simulink model "Assignment_2_3K04"  (R2022b)
settings: Solver=FixedStepAuto  StartTime=0.0  StopTime=1  FixedStep=1e-3  RelTol=1e-3  EnableMultiTasking=on
undefined symbols (not defined in the file): A0, A1, D0, D1, D10, D11, D12, D13, D2, D3, D4, D5, D6, D7, D8, D9, PTA0, PTA1, PTA2, PTB2, PTB23, PTB3, PTB9, PTC16, PTC17, PTC2, PTC3, PTC4, PTD0, PTD1, PTD2, PTD3
libraries: frdmk64flib x19, dspstat3 x1
settings Model: ExtModeTrigDuration=5  Creator=Stephen Oh  LastModifiedBy=Mehak
settings SolverCC: AlgebraicLoopSolver=TrustRegion
settings OptimizationCC: EnhancedBackFolding=on  PassReuseOutputArgsAs=Individual arguments  ZeroExternalMemoryAtStartup=off  ZeroInternalMemoryAtStartup=off  MaxStackSize=64  OptimizeBlockOrder=speed  DifferentSizesBufferReuse=on  OptimizationCustomize=off  EfficientTunableParamExpr=on
settings DebuggingCC: ParameterTunabilityLossMsg=error  UnconnectedInputMsg=warning  UnconnectedOutputMsg=warning  UnconnectedLineMsg=warning  SFMachineParentedDataDiag=warning
settings HardwareCC: ProdBitPerPointer=32  ProdBitPerSizeT=32  ProdBitPerPtrDiffT=32  ProdLargestAtomicInteger=Long  ProdLargestAtomicFloat=Double  ProdWordSize=32  ProdHWDeviceType=ARM Compatible->ARM Cortex
settings ModelReferenceCC: EnableRefExpFcnMdlSchedulingChecks=on
settings SFSimCC: MATLABDynamicMemAlloc=off
settings RTWCC: Description=Embedded Coder  SystemTargetFile=ert.tlc  HardwareBoard=NXP FRDM-K64F  TLCOptions="-aInlineSetEventsForThisBaseRateFcn=TLC_FALSE -aSuppressMultiTaskScheduler=TLC_FALSE  -aRateBasedStepFcn=0"  TemplateMakefile=ert_default_tmf  Toolchain=GNU Tools for ARM Embedded Processors
settings CodeAppCC: ForceParamTrailComments=on  IgnoreCustomStorageClasses=off  OperatorAnnotations=on  SimulinkDataObjDesc=on  SFDataObjDesc=on  InsertBlockDesc=on

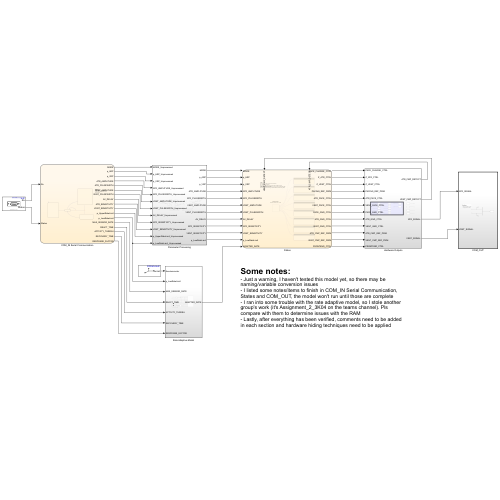
[thumbnail: Simulink's stored preview of the top-level diagram]
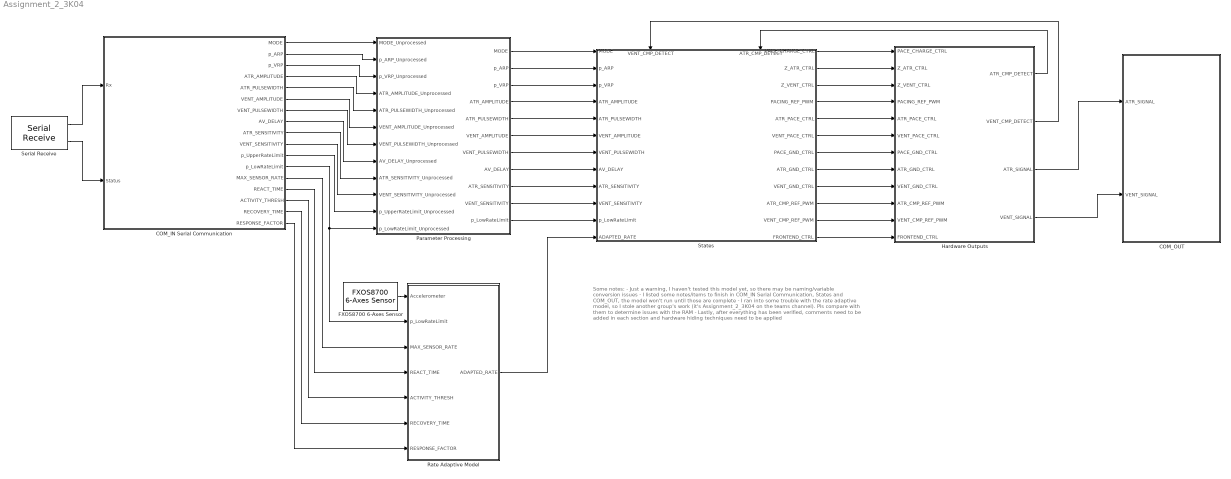
== system Assignment_2_3K04 ==
  note: Some notes:
      | - Just a warning, I haven't tested this model yet, so there may be naming/variable conversion issues
      | - I listed some notes/items to finish in COM_IN Serial Communication, States and COM_OUT, the model won't run until those are complete
      | - I ran into some trouble with the rate adaptive model, so I stole another group's work (it's Assignment_2_3K04 on the teams channel). Pls compare with them to determine issues with the RAM
      | - Lastly, after everything has been verified, comments need to be added in each section and hardware hiding techniques need to be applied
  " States" : Stateflow chart  TreatAsAtomicUnit=on
      settings: PortSchema="{\"entries\":[{\"content\":{\"sides\":[{\"content\":{\"connectorIds\":[\"In1\",\"In4\",\"In5\",\"In6\",\"In7\",\"In11\",\"In12\",\"In14\",\"In9\",\"In10\",\"In8\",\"In13\"]},\"type\":\"ConnectorPlacement.EquallySpacedRectSide\",\"uuid\":\"15e03f69-5c25-4f3e-b3fb-d71978e552f4\"},{\"content\":{\"connectorIds\":[\"Out7\",\"Out4\",\"Out5\",\"Out8\",\"Out9\",\"Out3\",\"Out6\",\"Out1\",\"Out2\",\"Out10\",\"Out12\",\"Out11\"],\"side\":\"RIGHT\"},\"type\":\"ConnectorPlacement.EquallySpacedRectSide\",\"uuid\":\"02171bf1-edb1-4b01-9e56-a8642c556ed6\"},{\"content\":{\"connectorIds\":[\"In3\",\"In2\"],\"side\":\"TOP\"},\"type\":\"ConnectorPlacement.EquallySpacedRectSide\",\"uuid\":\"cc6b5506-3435-4740-9e3f-4dfe15d30bff\"}]},\"type\":\"ConnectorPlacement.EquallySpacedConnector\",\"uuid\":\"0ad55da7-1e65-48d0-a0a4-2620ffa94320\"}],\"packageUris\":[\"http://schema.mathworks.com/mf0/Connector/R2020b\"],\"version\":\"1.0\"}"
  COM_IN Serial Communication : Stateflow chart  TreatAsAtomicUnit=on
      settings: PortSchema="{\"entries\":[{\"content\":{\"sides\":[{\"content\":{\"connectorIds\":[\"In1\",\"In2\"]},\"type\":\"ConnectorPlacement.EquallySpacedRectSide\",\"uuid\":\"22fa9edc-2a49-4280-8e8e-0842a45ddb47\"},{\"content\":{\"connectorIds\":[\"Out1\",\"Out2\",\"Out5\",\"Out6\",\"Out9\",\"Out7\",\"Out8\",\"Out11\",\"Out17\",\"Out12\",\"Out4\",\"Out3\",\"Out10\",\"Out13\",\"Out14\",\"Out16\",\"Out15\"],\"side\":\"RIGHT\"},\"type\":\"ConnectorPlacement.EquallySpacedRectSide\",\"uuid\":\"653d204d-01e6-4b1d-8e7b-47ebaddcd032\"},{\"content\":{\"connectorIds\":[],\"side\":\"TOP\"},\"type\":\"ConnectorPlacement.EquallySpacedRectSide\",\"uuid\":\"5fb759fd-937e-492d-8a65-272e5a7048d8\"}]},\"type\":\"ConnectorPlacement.EquallySpacedConnector\",\"uuid\":\"8ef65fa3-58c0-4e1e-983b-59a6af0cca9a\"}],\"packageUris\":[\"http://schema.mathworks.com/mf0/Connector/R2020b\"],\"version\":\"1.0\"}"
  COM_OUT : Subsystem  TreatAsAtomicUnit=on
  FXOS8700 6-Axes Sensor : frdmk64flib/FXOS8700 6-Axes Sensor  Activesensor=Accelerometer only  ODR=800Hz  HybridODR=400Hz  Accelfullrange=-4g to +4g  SampleTime=-1
  Hardware Outputs : Subsystem
  Parameter Processing : Subsystem
  Rate Adaptive Model : Subsystem
  Serial Receive : frdmk64flib/Serial Receive  SCIModule=0  Baudrate=uint32(9600)  Parity=None  StopBits=1  HardwareFlowControl=None  ByteOrder=LittleEndian  DataType=uint8  DataLength=34  BlockingMode=off  OutputStatus=on  SampleTime=0.1
  wires:
  " States"/7(PACE_CHARGE_CTRL) -> Hardware Outputs/1(PACE_CHARGE_CTRL)
  " States"/4(Z_ATR_CTRL) -> Hardware Outputs/2(Z_ATR_CTRL)
  " States"/5(Z_VENT_CTRL) -> Hardware Outputs/3(Z_VENT_CTRL)
  " States"/8(PACING_REF_PWM) -> Hardware Outputs/4(PACING_REF_PWM)
  " States"/9(ATR_PACE_CTRL) -> Hardware Outputs/5(ATR_PACE_CTRL)
  " States"/3(VENT_PACE_CTRL) -> Hardware Outputs/6(VENT_PACE_CTRL)
  " States"/6(PACE_GND_CTRL) -> Hardware Outputs/7(PACE_GND_CTRL)
  " States"/1(ATR_GND_CTRL) -> Hardware Outputs/8(ATR_GND_CTRL)
  " States"/2(VENT_GND_CTRL) -> Hardware Outputs/9(VENT_GND_CTRL)
  " States"/10(ATR_CMP_REF_PWM) -> Hardware Outputs/10(ATR_CMP_REF_PWM)
  " States"/12(VENT_CMP_REF_PWM) -> Hardware Outputs/11(VENT_CMP_REF_PWM)
  " States"/11(FRONTEND_CTRL) -> Hardware Outputs/12(FRONTEND_CTRL)
  Serial Receive/1 -> COM_IN Serial Communication/1(Rx)
  Serial Receive/2 -> COM_IN Serial Communication/2(Status)
  Hardware Outputs/1(ATR_CMP_DETECT) -> " States"/2(ATR_CMP_DETECT)
  Hardware Outputs/2(VENT_CMP_DETECT) -> " States"/3(VENT_CMP_DETECT)
  FXOS8700 6-Axes Sensor/1 -> Rate Adaptive Model/1(Accelerometer)
  COM_IN Serial Communication/3(p_LowRateLimit) -> Rate Adaptive Model/2(p_LowRateLimit), Parameter Processing/12(p_LowRateLimit_Unprocessed)
  COM_IN Serial Communication/10(MAX_SENSOR_RATE) -> Rate Adaptive Model/3(MAX_SENSOR_RATE)
  COM_IN Serial Communication/13(REACT_TIME) -> Rate Adaptive Model/4(REACT_TIME)
  COM_IN Serial Communication/14(ACTIVITY_THRESH) -> Rate Adaptive Model/5(ACTIVITY_THRESH)
  COM_IN Serial Communication/15(RESPONSE_FACTOR) -> Rate Adaptive Model/7(RESPONSE_FACTOR)
  COM_IN Serial Communication/16(RECOVERY_TIME) -> Rate Adaptive Model/6(RECOVERY_TIME)
  COM_IN Serial Communication/4(p_UpperRateLimit) -> Parameter Processing/11(p_UpperRateLimit_Unprocessed)
  COM_IN Serial Communication/17(ATR_SENSITIVITY) -> Parameter Processing/9(ATR_SENSITIVITY_Unprocessed)
  COM_IN Serial Communication/12(VENT_SENSITIVITY) -> Parameter Processing/10(VENT_SENSITIVITY_Unprocessed)
  COM_IN Serial Communication/6(ATR_AMPLITUDE) -> Parameter Processing/4(ATR_AMPLITUDE_Unprocessed)
  COM_IN Serial Communication/7(VENT_AMPLITUDE) -> Parameter Processing/6(VENT_AMPLITUDE_Unprocessed)
  COM_IN Serial Communication/1(MODE) -> Parameter Processing/1(MODE_Unprocessed)
  COM_IN Serial Communication/2(p_ARP) -> Parameter Processing/2(p_ARP_Unprocessed)
  COM_IN Serial Communication/5(p_VRP) -> Parameter Processing/3(p_VRP_Unprocessed)
  COM_IN Serial Communication/9(ATR_PULSEWIDTH) -> Parameter Processing/5(ATR_PULSEWIDTH_Unprocessed)
  COM_IN Serial Communication/8(VENT_PULSEWIDTH) -> Parameter Processing/7(VENT_PULSEWIDTH_Unprocessed)
  COM_IN Serial Communication/11(AV_DELAY) -> Parameter Processing/8(AV_DELAY_Unprocessed)
  Parameter Processing/1(MODE) -> " States"/1(MODE)
  Parameter Processing/2(p_ARP) -> " States"/4(p_ARP)
  Parameter Processing/3(p_VRP) -> " States"/5(p_VRP)
  Parameter Processing/11(p_LowRateLimit) -> " States"/8(p_LowRateLimit)
  Parameter Processing/10(VENT_SENSITIVITY) -> " States"/10(VENT_SENSITIVITY)
  Parameter Processing/9(ATR_SENSITIVITY) -> " States"/9(ATR_SENSITIVITY)
  Parameter Processing/4(ATR_AMPLITUDE) -> " States"/6(ATR_AMPLITUDE)
  Parameter Processing/5(ATR_PULSEWIDTH) -> " States"/7(ATR_PULSEWIDTH)
  Parameter Processing/6(VENT_AMPLITUDE) -> " States"/11(VENT_AMPLITUDE)
  Parameter Processing/7(VENT_PULSEWIDTH) -> " States"/12(VENT_PULSEWIDTH)
  Rate Adaptive Model/1(ADAPTED_RATE) -> " States"/13(ADAPTED_RATE)
  Parameter Processing/8(AV_DELAY) -> " States"/14(AV_DELAY)
  Hardware Outputs/3(ATR_SIGNAL) -> COM_OUT/1(ATR_SIGNAL)
  Hardware Outputs/4(VENT_SIGNAL) -> COM_OUT/2(VENT_SIGNAL)

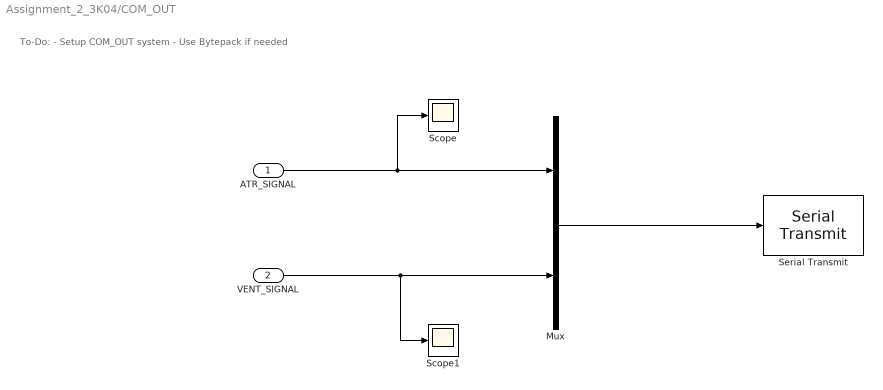
== system Assignment_2_3K04/COM_OUT ==
  note: To-Do:
      | - Setup COM_OUT system
      | - Use Bytepack if needed
  ATR_SIGNAL : Inport  OutDataTypeStr=double
  VENT_SIGNAL : Inport  Port=2  OutDataTypeStr=double
  Mux : Mux  Inputs=2
  Scope : Scope
  Scope1 : Scope
  Serial Transmit : frdmk64flib/Serial Transmit  SCIModule=0  Baudrate=uint32(9600)  Parity=None  StopBits=1  HardwareFlowControl=None  ByteOrder=LittleEndian  BlockingMode=on  OutputStatus=off
  wires:
  ATR_SIGNAL/1 -> Scope/1, Mux/1
  Mux/1 -> Serial Transmit/1
  VENT_SIGNAL/1 -> Scope1/1, Mux/2

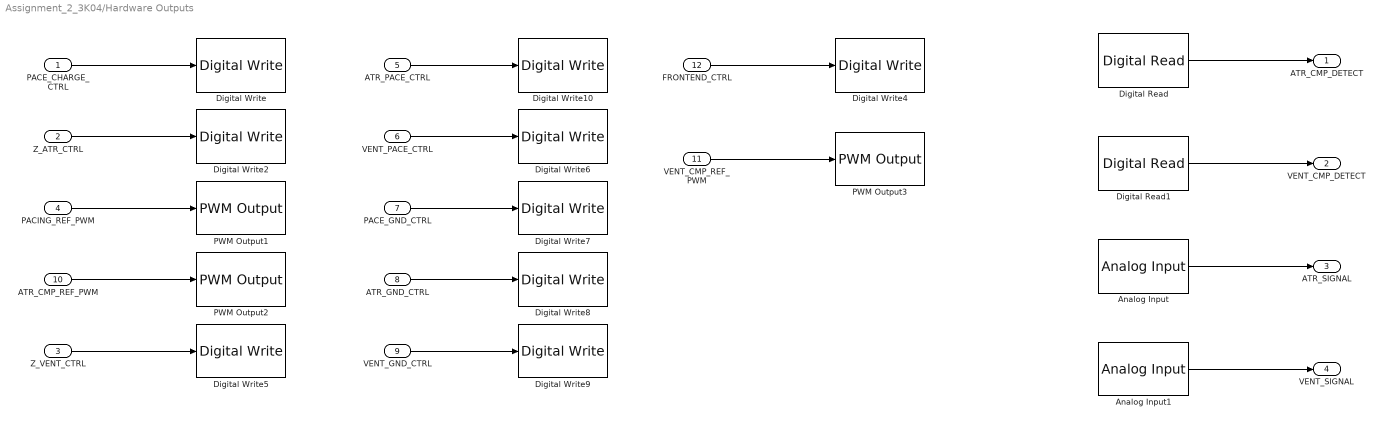
== system Assignment_2_3K04/Hardware Outputs ==
  PACE_CHARGE_CTRL : Inport
  Z_ATR_CTRL : Inport  Port=2
  Z_VENT_CTRL : Inport  Port=3
  PACING_REF_PWM : Inport  Port=4
  ATR_PACE_CTRL : Inport  Port=5
  VENT_PACE_CTRL : Inport  Port=6
  PACE_GND_CTRL : Inport  Port=7
  ATR_GND_CTRL : Inport  Port=8
  VENT_GND_CTRL : Inport  Port=9
  ATR_CMP_REF_PWM : Inport  Port=10
  VENT_CMP_REF_PWM : Inport  Port=11
  FRONTEND_CTRL : Inport  Port=12
  Analog Input : frdmk64flib/Analog Input  Whichpin=PTB2 (A0)  SampleTime=-1
  Analog Input1 : frdmk64flib/Analog Input  Whichpin=PTB3 (A1)  SampleTime=-1
  Digital Read : frdmk64flib/Digital Read  Whichpin=PTC16 (D0)  SampleTime=-1
  Digital Read1 : frdmk64flib/Digital Read  Whichpin=PTC17 (D1)  SampleTime=-1
  Digital Write : frdmk64flib/Digital Write  Whichpin=PTB9 (D2)
  Digital Write10 : frdmk64flib/Digital Write  Whichpin=PTA0 (D8)
  Digital Write2 : frdmk64flib/Digital Write  Whichpin=PTB23 (D4)
  Digital Write4 : frdmk64flib/Digital Write  Whichpin=PTD1 (D13)
  Digital Write5 : frdmk64flib/Digital Write  Whichpin=PTC3 (D7)
  Digital Write6 : frdmk64flib/Digital Write  Whichpin=PTC4 (D9)
  Digital Write7 : frdmk64flib/Digital Write  Whichpin=PTD0 (D10)
  Digital Write8 : frdmk64flib/Digital Write  Whichpin=PTD2 (D11)
  Digital Write9 : frdmk64flib/Digital Write  Whichpin=PTD3 (D12)
  PWM Output1 : frdmk64flib/PWM Output  Whichpin=PTA2 (D5)  InitialFrequency=2000  InitialDutyCycle=0
  PWM Output2 : frdmk64flib/PWM Output  Whichpin=PTC2 (D6)  InitialFrequency=2000  InitialDutyCycle=0
  PWM Output3 : frdmk64flib/PWM Output  Whichpin=PTA1 (D3)  InitialFrequency=2000  InitialDutyCycle=0
  ATR_CMP_DETECT : Outport
  VENT_CMP_DETECT : Outport  Port=2
  ATR_SIGNAL : Outport  Port=3  OutDataTypeStr=double
  VENT_SIGNAL : Outport  Port=4  OutDataTypeStr=double
  wires:
  ATR_GND_CTRL/1 -> Digital Write8/1
  Z_ATR_CTRL/1 -> Digital Write2/1
  VENT_PACE_CTRL/1 -> Digital Write6/1
  PACING_REF_PWM/1 -> PWM Output1/1
  VENT_GND_CTRL/1 -> Digital Write9/1
  PACE_GND_CTRL/1 -> Digital Write7/1
  FRONTEND_CTRL/1 -> Digital Write4/1
  PACE_CHARGE_CTRL/1 -> Digital Write/1
  Z_VENT_CTRL/1 -> Digital Write5/1
  ATR_CMP_REF_PWM/1 -> PWM Output2/1
  ATR_PACE_CTRL/1 -> Digital Write10/1
  VENT_CMP_REF_PWM/1 -> PWM Output3/1
  Digital Read/1 -> ATR_CMP_DETECT/1
  Digital Read1/1 -> VENT_CMP_DETECT/1
  Analog Input/1 -> ATR_SIGNAL/1
  Analog Input1/1 -> VENT_SIGNAL/1

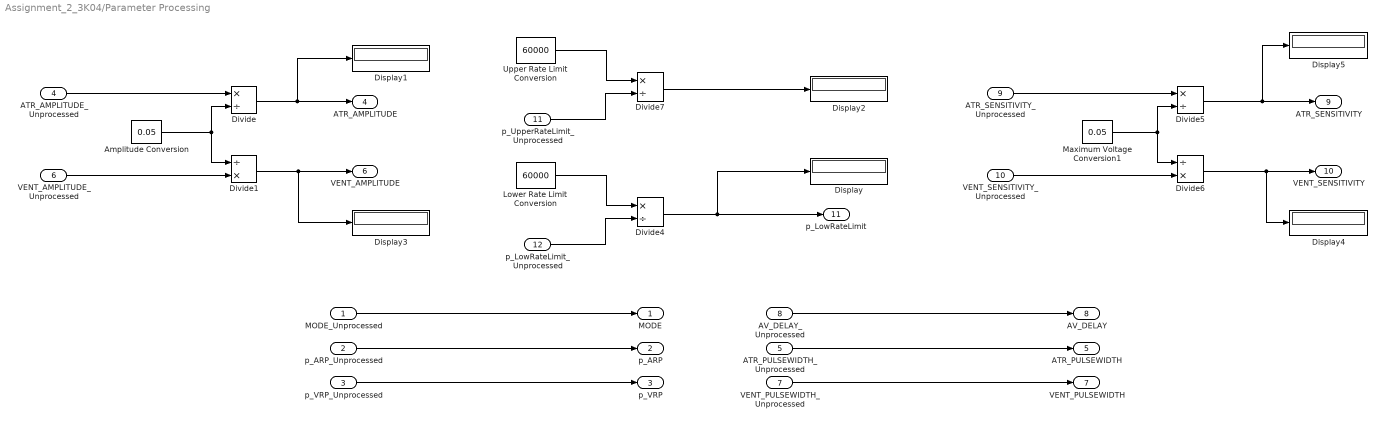
== system Assignment_2_3K04/Parameter Processing ==
  MODE_Unprocessed : Inport  OutDataTypeStr=single
  p_ARP_Unprocessed : Inport  Port=2  OutDataTypeStr=single
  p_VRP_Unprocessed : Inport  Port=3  OutDataTypeStr=single
  ATR_AMPLITUDE_Unprocessed : Inport  Port=4  OutDataTypeStr=single
  ATR_PULSEWIDTH_Unprocessed : Inport  Port=5  OutDataTypeStr=single
  VENT_AMPLITUDE_Unprocessed : Inport  Port=6  OutDataTypeStr=single
  VENT_PULSEWIDTH_Unprocessed : Inport  Port=7  OutDataTypeStr=single
  AV_DELAY_Unprocessed : Inport  Port=8  OutDataTypeStr=single
  ATR_SENSITIVITY_Unprocessed : Inport  Port=9  OutDataTypeStr=single
  VENT_SENSITIVITY_Unprocessed : Inport  Port=10  OutDataTypeStr=single
  p_UpperRateLimit_Unprocessed : Inport  Port=11
  p_LowRateLimit_Unprocessed : Inport  Port=12
  Amplitude Conversion : Constant  Value=0.05
  Display{,1..5} (6 alike) : Display
  Divide : Product  Inputs=*/  OutDataTypeStr=uint8
  Divide1 : Product  Inputs=/*  OutDataTypeStr=uint8
  Divide4 : Product  Inputs=*/  OutDataTypeStr=Inherit: Keep MSB  RndMeth=Nearest
  Divide5 : Product  Inputs=*/  OutDataTypeStr=uint8
  Divide6 : Product  Inputs=/*  OutDataTypeStr=uint8
  Divide7 : Product  Inputs=*/  OutDataTypeStr=Inherit: Keep MSB  RndMeth=Nearest
  Lower Rate Limit Conversion : Constant  Value=60000
  Maximum Voltage Conversion1 : Constant  Value=0.05
  Upper Rate Limit Conversion : Constant  Value=60000
  MODE : Outport
  p_ARP : Outport  Port=2
  p_VRP : Outport  Port=3
  ATR_AMPLITUDE : Outport  Port=4  OutDataTypeStr=uint8
  ATR_PULSEWIDTH : Outport  Port=5
  VENT_AMPLITUDE : Outport  Port=6  OutDataTypeStr=uint8
  VENT_PULSEWIDTH : Outport  Port=7
  AV_DELAY : Outport  Port=8
  ATR_SENSITIVITY : Outport  Port=9  OutDataTypeStr=uint8
  VENT_SENSITIVITY : Outport  Port=10  OutDataTypeStr=uint8
  p_LowRateLimit : Outport  Port=11
  wires:
  Amplitude Conversion/1 -> Divide1/1, Divide/2
  ATR_AMPLITUDE_Unprocessed/1 -> Divide/1
  VENT_AMPLITUDE_Unprocessed/1 -> Divide1/2
  Divide/1 -> Display1/1, ATR_AMPLITUDE/1
  Divide1/1 -> Display3/1, VENT_AMPLITUDE/1
  Divide6/1 -> Display4/1, VENT_SENSITIVITY/1
  Maximum Voltage Conversion1/1 -> Divide6/1, Divide5/2
  ATR_SENSITIVITY_Unprocessed/1 -> Divide5/1
  Divide5/1 -> Display5/1, ATR_SENSITIVITY/1
  VENT_SENSITIVITY_Unprocessed/1 -> Divide6/2
  Divide4/1 -> p_LowRateLimit/1, Display/1
  p_LowRateLimit_Unprocessed/1 -> Divide4/2
  Lower Rate Limit Conversion/1 -> Divide4/1
  Divide7/1 -> Display2/1
  Upper Rate Limit Conversion/1 -> Divide7/1
  p_UpperRateLimit_Unprocessed/1 -> Divide7/2
  MODE_Unprocessed/1 -> MODE/1
  p_ARP_Unprocessed/1 -> p_ARP/1
  p_VRP_Unprocessed/1 -> p_VRP/1
  VENT_PULSEWIDTH_Unprocessed/1 -> VENT_PULSEWIDTH/1
  AV_DELAY_Unprocessed/1 -> AV_DELAY/1
  ATR_PULSEWIDTH_Unprocessed/1 -> ATR_PULSEWIDTH/1

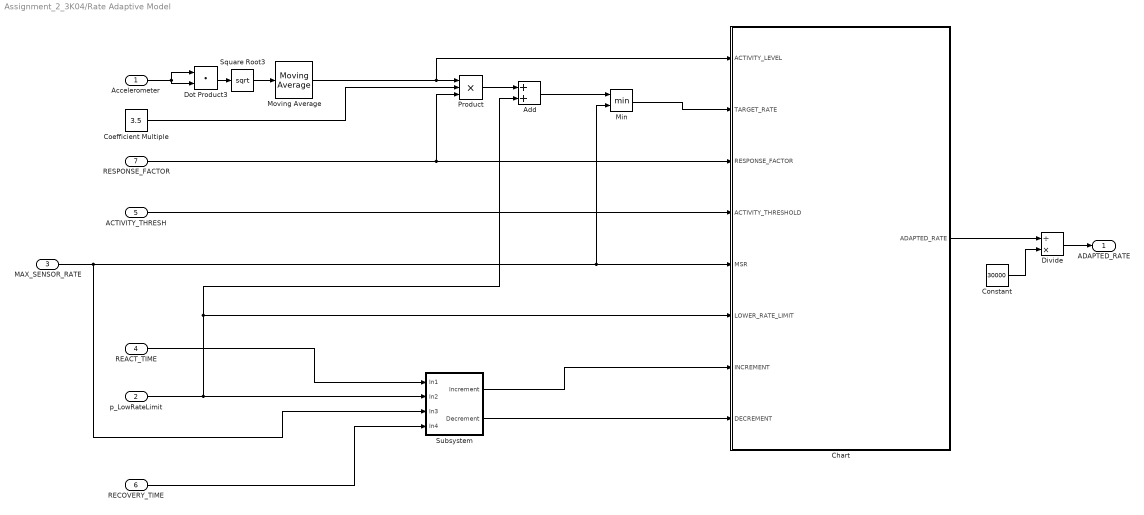
== system Assignment_2_3K04/Rate Adaptive Model ==
  Accelerometer : Inport
  p_LowRateLimit : Inport  Port=2
  MAX_SENSOR_RATE : Inport  Port=3
  REACT_TIME : Inport  Port=4
  ACTIVITY_THRESH : Inport  Port=5
  RECOVERY_TIME : Inport  Port=6
  RESPONSE_FACTOR : Inport  Port=7
  Add : Sum
  Chart : Stateflow chart  TreatAsAtomicUnit=on
      settings: PortSchema="{\"entries\":[{\"content\":{\"sides\":[{\"content\":{\"connectorIds\":[\"In1\",\"In3\",\"In2\",\"In6\",\"In8\",\"In7\",\"In4\",\"In5\"]},\"type\":\"ConnectorPlacement.EquallySpacedRectSide\",\"uuid\":\"efebee7e-2c09-4b25-ba04-904f72c011ed\"},{\"content\":{\"connectorIds\":[\"Out1\"],\"side\":\"RIGHT\"},\"type\":\"ConnectorPlacement.EquallySpacedRectSide\",\"uuid\":\"6322cc63-1b7a-423a-b49b-7b27e71e0c32\"},{\"content\":{\"connectorIds\":[],\"side\":\"TOP\"},\"type\":\"ConnectorPlacement.EquallySpacedRectSide\",\"uuid\":\"daf2dbd4-7676-46e9-bb01-958bd0e2e14e\"}]},\"type\":\"ConnectorPlacement.EquallySpacedConnector\",\"uuid\":\"43c3c7b3-b94c-45f5-b310-1a430cfb2b71\"}],\"packageUris\":[\"http://schema.mathworks.com/mf0/Connector/19700101\"],\"version\":\"1.0\"}"
  Coefficient Multiple : Constant  Value=3.5
  Constant : Constant  Value=30000
  Divide : Product  Inputs=/*
  Dot Product3 : DotProduct  OutDataTypeStr=Inherit: Inherit via internal rule
  Min : MinMax  Inputs=2
  Moving Average : dspstat3/Moving Average  Method=Sliding window  ForgettingFactorPort=off  SpecifyWindowLength=on  WindowLength=500  OverlapLength=499  AllowArbitraryInputLength=off  ForgettingFactor=0.9  SimulateUsing=Code generation
  Product : Product  Inputs=3
  Square Root3 : Sqrt
  Subsystem : Subsystem
  ADAPTED_RATE : Outport
  wires:
  RECOVERY_TIME/1 -> Subsystem/4(In4)
  MAX_SENSOR_RATE/1 -> Subsystem/3(In3), Min/2, Chart/8(MSR)
  Subsystem/1(Increment) -> Chart/4(INCREMENT)
  ACTIVITY_THRESH/1 -> Chart/6(ACTIVITY_THRESHOLD)
  RESPONSE_FACTOR/1 -> Product/3, Chart/2(RESPONSE_FACTOR)
  p_LowRateLimit/1 -> Subsystem/2(In2), Chart/7(LOWER_RATE_LIMIT), Add/2
  Add/1 -> Min/1
  Product/1 -> Add/1
  Min/1 -> Chart/3(TARGET_RATE)
  REACT_TIME/1 -> Subsystem/1(In1)
  Subsystem/2(Decrement) -> Chart/5(DECREMENT)
  Chart/1(ADAPTED_RATE) -> Divide/1
  Coefficient Multiple/1 -> Product/2
  Divide/1 -> ADAPTED_RATE/1
  Constant/1 -> Divide/2
  Moving Average/1 -> Chart/1(ACTIVITY_LEVEL), Product/1
  Square Root3/1 -> Moving Average/1
  Dot Product3/1 -> Square Root3/1
  Accelerometer/1 -> Dot Product3/1, Dot Product3/2

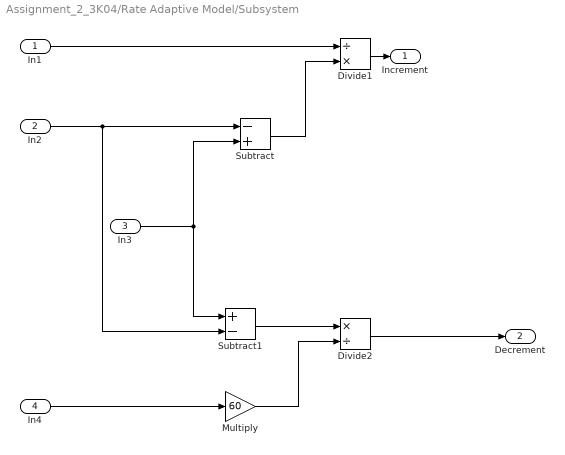
== system Assignment_2_3K04/Rate Adaptive Model/Subsystem ==
  In1 : Inport
  In2 : Inport  Port=2
  In3 : Inport  Port=3
  In4 : Inport  Port=4
  Divide1 : Product  Inputs=/*  OutDataTypeStr=uint8  RndMeth=Ceiling
  Divide2 : Product  Inputs=*/  OutDataTypeStr=uint8  RndMeth=Ceiling  SaturateOnIntegerOverflow=on
  Multiply : Gain  Gain=60
  Subtract : Sum  Inputs=-+
  Subtract1 : Sum  Inputs=+-
  Increment : Outport
  Decrement : Outport  Port=2
  wires:
  Multiply/1 -> Divide2/2
  In2/1 -> Subtract1/2, Subtract/1
  In3/1 -> Subtract/2, Subtract1/1
  Divide1/1 -> Increment/1
  In1/1 -> Divide1/1
  Subtract1/1 -> Divide2/1
  Subtract/1 -> Divide1/2
  In4/1 -> Multiply/1
  Divide2/1 -> Decrement/1

== stateflow chart Assignment_2_3K04/COM_IN Serial Communication ==
  state SET_PARAM
    % Uses serial input to assign values to the parameters
    entry:
    MODE = Rx();
    p_LowRateLimit = Rx();
    p_UpperRateLimit = Rx();
    ATR_AMPLITUDE = Rx();
    VENT_AMPLITUDE = Rx();
    ATR_PULSEWIDTH = Rx();
    VENT_PULSEWIDTH = Rx();
    p_ARP = Rx();
    p_VRP = Rx();
    ATR_SENSITIVITY = Rx();
    VENT_SENSITIVITY = Rx();
    MAX_SENSOR_RATE = Rx();
    RECOVERY_TIME = Rx();
    REACT_TIME = Rx();
    RESPONSE_FACTOR = Rx();
    ACTIVITY_THRESH = Rx();
    AV_DELAY = Rx();
  note: To-Do:
      | - Set number of transmitted bytes
      | - Update SET_PARAM with values
      | - Verify Fuction
  state INITIAL
    % Set the initial values of parameters
    entry:
    MODE = 1;
    p_ARP = 250;
    p_VRP = 320;
    p_LowRateLimit = 60;
    p_UpperRateLimit = 120;
    MAX_SENSOR_RATE = 120;
    ATR_AMPLITUDE = 3.5;
    ATR_PULSEWIDTH = 1;
    VENT_AMPLITUDE = 3.5;
    VENT_PULSEWIDTH = 1;
    AV_DELAY = 150;
    ATR_SENSITIVITY = 4;
    VENT_SENSITIVITY = 4;
    REACT_TIME = 30;
    ACTIVITY_THRESH = 1.1;
    RESPONSE_FACTOR = 8;
    RECOVERY_TIME = 5;
  state STANDBY
    % Wait for COM
  state ECHO_PARAM
    % Sends back the current value of the parameters
    entry:
    send_params()
  (default) -> INITIAL
  SET_PARAM -> STANDBY
  (junction 13) -> SET_PARAM [order 1] : [Rx(2) == hex2dec('55')]
  (junction 12) -> STANDBY [order 2]
  INITIAL -> STANDBY
  STANDBY -> (junction 12) : [Status==0]
  (junction 12) -> (junction 13) [order 1] : [Rx(1) == hex2dec('16')]
  (junction 13) -> ECHO_PARAM [order 2] : [Rx(2) == hex2dec('22')]
  ECHO_PARAM -> STANDBY
  data: Rx input uint8; Status input uint8; MODE output uint8; p_ARP output uint16; p_LowRateLimit output uint8; p_UpperRateLimit output uint8; p_VRP output uint16; ATR_AMPLITUDE output single; VENT_AMPLITUDE output single; VENT_PULSEWIDTH output uint8; ATR_PULSEWIDTH output uint8; MAX_SENSOR_RATE output uint8; AV_DELAY output uint16; VENT_SENSITIVITY output single; REACT_TIME output uint8; ACTIVITY_THRESH output single; RESPONSE_FACTOR output uint8; RECOVERY_TIME output uint8; ATR_SENSITIVITY output single

== stateflow chart Assignment_2_3K04/Rate Adaptive Model/Chart ==
  state RateSelect
    entry:
    ADAPTED_RATE = LOWER_RATE_LIMIT
  state Increment
    entry:
    ADAPTED_RATE = ADAPTED_RATE + INCREMENT
  state TargetRateAchieved
  state Decrement
    entry:
    ADAPTED_RATE = ADAPTED_RATE - DECREMENT
  Increment -> Increment [order 2] : after(1000, msec) [ACTIVITY_LEVEL > ACTIVITY_THRESHOLD]
  (default) -> RateSelect
  Increment -> TargetRateAchieved [order 1] : [ADAPTED_RATE >= TARGET_RATE ]
  RateSelect -> Increment [order 1] : [ACTIVITY_LEVEL > ACTIVITY_THRESHOLD]
  RateSelect -> RateSelect [order 2] : [ACTIVITY_LEVEL < ACTIVITY_THRESHOLD]
  Decrement -> RateSelect [order 3] : [ADAPTED_RATE <= LOWER_RATE_LIMIT]
  Decrement -> Increment [order 1] : after(1000, msec) [ACTIVITY_LEVEL > ACTIVITY_THRESHOLD]
  Increment -> Decrement [order 3] : after(1000, msec) [ACTIVITY_LEVEL < ACTIVITY_THRESHOLD]
  TargetRateAchieved -> Decrement : [ACTIVITY_LEVEL < ACTIVITY_THRESHOLD]
  Decrement -> Decrement [order 2] : after(1000, msec) [ACTIVITY_LEVEL < ACTIVITY_THRESHOLD]
  data: ACTIVITY_LEVEL input; RESPONSE_FACTOR input; ADAPTED_RATE output; TARGET_RATE input; INCREMENT input; DECREMENT input; ACTIVITY_THRESHOLD input; LOWER_RATE_LIMIT input; MSR input

== stateflow chart Assignment_2_3K04/ States ==
  state AOO [group]
    state Charging
      entry:
      %charging capacitor C22
      ATR_PACE_CTRL = 0;
      VENT_PACE_CTRL = 0;
      PACING_REF_PWM = ATR_AMPLITUDE;
      PACE_CHARGE_CTRL = 1;
    state Pacing
      entry:
      %charge release of capacitor C22 into C21
      PACE_CHARGE_CTRL = 0;
      PACE_GND_CTRL = 1;
      ATR_PACE_CTRL = 1;
      ATR_GND_CTRL = 0;
      Z_ATR_CTRL = 0;
      Z_VENT_CTRL = 0;
      VENT_GND_CTRL = 0;
      VENT_PACE_CTRL = 0;
    state Discharging
      entry:
      %charging release of capacitor C21 to gnd
      PACE_GND_CTRL = 1;
      VENT_PACE_CTRL = 0;
      Z_ATR_CTRL = 0;
      Z_VENT_CTRL = 0;
      ATR_PACE_CTRL = 0;
      ATR_GND_CTRL = 1;
      VENT_GND_CTRL = 0;
    AOO.Pacing -> AOO.Discharging : after(ATR_PULSEWIDTH, msec)
    AOO.Charging -> AOO.Pacing : after(p_LowRateLimit, msec)
    AOO.Discharging -> AOO.Charging
  note: To-Do:
      | - Verify that AOO, VOO, AAI, VVI work as intended
      | - Then test AOOR and VOOR
      | - If the previous two cases function as intended, test AAIR and VVIR
      | - If AAIR and VVIR don't work, subtract p_ARP/p_VRP from ADAPTED_RATE
      | - Finally, add comments + organize
      | - If there is enough time remaining, implement DDDR (else delete AV_DELAY)
  state VOO [group]
    state Pacing
      entry:
      %charge release of capacitor C22 into C21
      PACE_CHARGE_CTRL = 0;
      PACE_GND_CTRL = 1;
      ATR_PACE_CTRL = 0;
      ATR_GND_CTRL = 0;
      Z_ATR_CTRL = 0;
      Z_VENT_CTRL = 0;
      VENT_GND_CTRL = 0;
      VENT_PACE_CTRL = 1;
    state Discharging
      entry:
      %charging release of capacitor C21 to gnd
      PACE_GND_CTRL = 1;
      VENT_PACE_CTRL = 0;
      Z_ATR_CTRL = 0;
      Z_VENT_CTRL = 0;
      ATR_PACE_CTRL = 0;
      ATR_GND_CTRL = 0;
      VENT_GND_CTRL = 1;
    state Charging
      entry:
      %charging capacitor C22
      ATR_PACE_CTRL = 0;
      VENT_PACE_CTRL = 0;
      PACING_REF_PWM = VENT_AMPLITUDE;
      PACE_CHARGE_CTRL = 1;
    VOO.Pacing -> VOO.Discharging : after(VENT_PULSEWIDTH, msec)
    VOO.Charging -> VOO.Pacing : after(p_LowRateLimit, msec)
    VOO.Discharging -> VOO.Charging
  state AAI [group]
    state Pacing
      entry:
      %charging release of capacitor C21 to gnd
      PACE_CHARGE_CTRL = 0;
      PACE_GND_CTRL = 1;
      ATR_PACE_CTRL = 1;
      ATR_GND_CTRL = 0;
      Z_ATR_CTRL = 0;
      Z_VENT_CTRL = 0;
      VENT_GND_CTRL = 0;
      VENT_PACE_CTRL = 0;
    state Charging
      entry:
      % turn sensing ON
      FRONTEND_CTRL = 1;
      ATR_CMP_REF_PWM = ATR_SENSITIVITY;
      %charging capacitor C22
      PACING_REF_PWM = ATR_AMPLITUDE;
      PACE_CHARGE_CTRL = 1;
      VENT_PACE_CTRL = 0;
      ATR_PACE_CTRL = 0;
    note: Check for intrinsic pulse
    state Discharging
      entry:
      %charging release of capacitor C21 to gnd
      PACE_GND_CTRL = 1;
      VENT_PACE_CTRL = 0;
      ATR_PACE_CTRL = 0;
      Z_ATR_CTRL = 0;
      Z_VENT_CTRL = 0;
      ATR_GND_CTRL = 1;
      VENT_GND_CTRL = 0;
    (junction 150) -> AAI.Charging [order 1] : [ATR_CMP_DETECT == 1]
    AAI.Charging -> (junction 150) : after(p_ARP, msec)
    (junction 150) -> AAI.Pacing [order 2] : after(p_LowRateLimit, msec)
    AAI.Pacing -> AAI.Discharging : after(ATR_PULSEWIDTH, msec)
    AAI.Discharging -> AAI.Charging
  note: Mode Selection
  state VVI [group]
    state Pacing
      entry:
      %charging release of capacitor C21 to gnd
      PACE_CHARGE_CTRL = 0;
      PACE_GND_CTRL = 1;
      ATR_PACE_CTRL = 0;
      ATR_GND_CTRL = 0;
      Z_ATR_CTRL = 0;
      Z_VENT_CTRL = 0;
      VENT_GND_CTRL = 0;
      VENT_PACE_CTRL = 1;
    state Charging
      entry:
      % turn sensing ON
      FRONTEND_CTRL = 1;
      VENT_CMP_REF_PWM = VENT_SENSITIVITY;
      %charging capacitor C22
      PACING_REF_PWM = ATR_AMPLITUDE;
      PACE_CHARGE_CTRL = 1;
      VENT_PACE_CTRL = 0;
      ATR_PACE_CTRL = 0;
    note: Check for intrinsic pulse
    state Discharging
      entry:
      %charging release of capacitor C21 to gnd
      PACE_GND_CTRL = 1;
      VENT_PACE_CTRL = 0;
      ATR_PACE_CTRL = 0;
      Z_ATR_CTRL = 0;
      Z_VENT_CTRL = 0;
      ATR_GND_CTRL = 0;
      VENT_GND_CTRL = 1;
    (junction 155) -> VVI.Charging [order 1] : [VENT_CMP_DETECT == 1]
    (junction 155) -> VVI.Pacing [order 2] : after(p_LowRateLimit, msec)
    VVI.Charging -> (junction 155) : after(p_VRP, msec)
    VVI.Pacing -> VVI.Discharging : after(ATR_PULSEWIDTH, msec)
    VVI.Discharging -> VVI.Charging
  note: Conditional transition for the 4 modes
  state ModeSelect
  state AOOR [group]
    state Charging
      entry:
      %charging capacitor C22
      ATR_PACE_CTRL = 0;
      VENT_PACE_CTRL = 0;
      PACING_REF_PWM = ATR_AMPLITUDE;
      PACE_CHARGE_CTRL = 1;
    state Pacing
      entry:
      %charge release of capacitor C22 into C21
      PACE_CHARGE_CTRL = 0;
      PACE_GND_CTRL = 1;
      ATR_PACE_CTRL = 1;
      ATR_GND_CTRL = 0;
      Z_ATR_CTRL = 0;
      Z_VENT_CTRL = 0;
      VENT_GND_CTRL = 0;
      VENT_PACE_CTRL = 0;
    state Discharging
      entry:
      %charging release of capacitor C21 to gnd
      PACE_GND_CTRL = 1;
      VENT_PACE_CTRL = 0;
      Z_ATR_CTRL = 0;
      Z_VENT_CTRL = 0;
      ATR_PACE_CTRL = 0;
      ATR_GND_CTRL = 1;
      VENT_GND_CTRL = 0;
    AOOR.Pacing -> AOOR.Discharging : after(ATR_PULSEWIDTH, msec)
    AOOR.Charging -> AOOR.Pacing : after(ADAPTED_RATE, msec)
    AOOR.Discharging -> AOOR.Charging
  state VOOR [group]
    state Pacing
      entry:
      %charge release of capacitor C22 into C21
      PACE_CHARGE_CTRL = 0;
      PACE_GND_CTRL = 1;
      ATR_PACE_CTRL = 0;
      ATR_GND_CTRL = 0;
      Z_ATR_CTRL = 0;
      Z_VENT_CTRL = 0;
      VENT_GND_CTRL = 0;
      VENT_PACE_CTRL = 1;
    state Discharging
      entry:
      %charging release of capacitor C21 to gnd
      PACE_GND_CTRL = 1;
      VENT_PACE_CTRL = 0;
      Z_ATR_CTRL = 0;
      Z_VENT_CTRL = 0;
      ATR_PACE_CTRL = 0;
      ATR_GND_CTRL = 0;
      VENT_GND_CTRL = 1;
    state Charging
      entry:
      %charging capacitor C22
      ATR_PACE_CTRL = 0;
      VENT_PACE_CTRL = 0;
      PACING_REF_PWM = VENT_AMPLITUDE;
      PACE_CHARGE_CTRL = 1;
    VOOR.Pacing -> VOOR.Discharging : after(VENT_PULSEWIDTH, msec)
    VOOR.Charging -> VOOR.Pacing : after(ADAPTED_RATE, msec)
    VOOR.Discharging -> VOOR.Charging
  state AAIR [group]
    state Pacing
      entry:
      %charging release of capacitor C21 to gnd
      PACE_CHARGE_CTRL = 0;
      PACE_GND_CTRL = 1;
      ATR_PACE_CTRL = 1;
      ATR_GND_CTRL = 0;
      Z_ATR_CTRL = 0;
      Z_VENT_CTRL = 0;
      VENT_GND_CTRL = 0;
      VENT_PACE_CTRL = 0;
    state Charging
      entry:
      % turn sensing ON
      FRONTEND_CTRL = 1;
      ATR_CMP_REF_PWM = ATR_SENSITIVITY;
      %charging capacitor C22
      PACING_REF_PWM = ATR_AMPLITUDE;
      PACE_CHARGE_CTRL = 1;
      VENT_PACE_CTRL = 0;
      ATR_PACE_CTRL = 0;
    note: Check for intrinsic pulse
    state Discharging
      entry:
      %charging release of capacitor C21 to gnd
      PACE_GND_CTRL = 1;
      VENT_PACE_CTRL = 0;
      ATR_PACE_CTRL = 0;
      Z_ATR_CTRL = 0;
      Z_VENT_CTRL = 0;
      ATR_GND_CTRL = 1;
      VENT_GND_CTRL = 0;
    (junction 304) -> AAIR.Charging [order 1] : [ATR_CMP_DETECT == 1]
    AAIR.Charging -> (junction 304) : after(p_ARP, msec)
    (junction 304) -> AAIR.Pacing [order 2] : after(ADAPTED_RATE, msec)
    AAIR.Pacing -> AAIR.Discharging : after(ATR_PULSEWIDTH, msec)
    AAIR.Discharging -> AAIR.Charging
  state VVIR [group]
    state Pacing
      entry:
      %charging release of capacitor C21 to gnd
      PACE_CHARGE_CTRL = 0;
      PACE_GND_CTRL = 1;
      ATR_PACE_CTRL = 0;
      ATR_GND_CTRL = 0;
      Z_ATR_CTRL = 0;
      Z_VENT_CTRL = 0;
      VENT_GND_CTRL = 0;
      VENT_PACE_CTRL = 1;
    state Charging
      entry:
      % turn sensing ON
      FRONTEND_CTRL = 1;
      VENT_CMP_REF_PWM = VENT_SENSITIVITY;
      %charging capacitor C22
      PACING_REF_PWM = ATR_AMPLITUDE;
      PACE_CHARGE_CTRL = 1;
      VENT_PACE_CTRL = 0;
      ATR_PACE_CTRL = 0;
    note: Check for intrinsic pulse
    state Discharging
      entry:
      %charging release of capacitor C21 to gnd
      PACE_GND_CTRL = 1;
      VENT_PACE_CTRL = 0;
      ATR_PACE_CTRL = 0;
      Z_ATR_CTRL = 0;
      Z_VENT_CTRL = 0;
      ATR_GND_CTRL = 0;
      VENT_GND_CTRL = 1;
    (junction 284) -> VVIR.Charging [order 1] : [VENT_CMP_DETECT == 1]
    (junction 284) -> VVIR.Pacing [order 2] : after(ADAPTED_RATE, msec)
    VVIR.Charging -> (junction 284) : after(p_VRP, msec)
    VVIR.Pacing -> VVIR.Discharging : after(ATR_PULSEWIDTH, msec)
    VVIR.Discharging -> VVIR.Charging
  ModeSelect -> AOO.Charging [order 4] : [MODE == 0]
  ModeSelect -> VOO.Charging [order 6] : [MODE == 1]
  ModeSelect -> VVI.Charging [order 8] : [MODE == 3]
  ModeSelect -> AAI.Charging [order 7] : [MODE == 2]
  ModeSelect -> AOOR.Charging [order 5] : [MODE == 4]
  (default) -> ModeSelect
  ModeSelect -> VOOR.Charging [order 2] : [MODE == 5]
  ModeSelect -> AAIR.Charging [order 3] : [MODE == 6]
  ModeSelect -> VVIR.Charging [order 1] : [MODE == 7]
  data: ATR_GND_CTRL output; VENT_GND_CTRL output; VENT_PACE_CTRL output; Z_ATR_CTRL output; Z_VENT_CTRL output; PACE_GND_CTRL output; PACE_CHARGE_CTRL output; PACING_REF_PWM output; ATR_PACE_CTRL output; MODE input; ATR_CMP_REF_PWM output; FRONTEND_CTRL output; VENT_CMP_REF_PWM output; ATR_CMP_DETECT input; VENT_CMP_DETECT input; p_ARP input; p_VRP input; ATR_AMPLITUDE input; ATR_PULSEWIDTH input; p_LowRateLimit input; ATR_SENSITIVITY input; VENT_SENSITIVITY input; VENT_AMPLITUDE input; VENT_PULSEWIDTH input; ADAPTED_RATE input; AV_DELAY input
